simulink model "fft_filter"  (R2018a)
settings: Solver=VariableStepAuto  StartTime=0.0  StopTime=10  RelTol=1e-3
libraries: xbsIndex_r4 x6
settings Model: Creator=ESPINO NOTEBOOK  LastModifiedBy=ESPINO NOTEBOOK

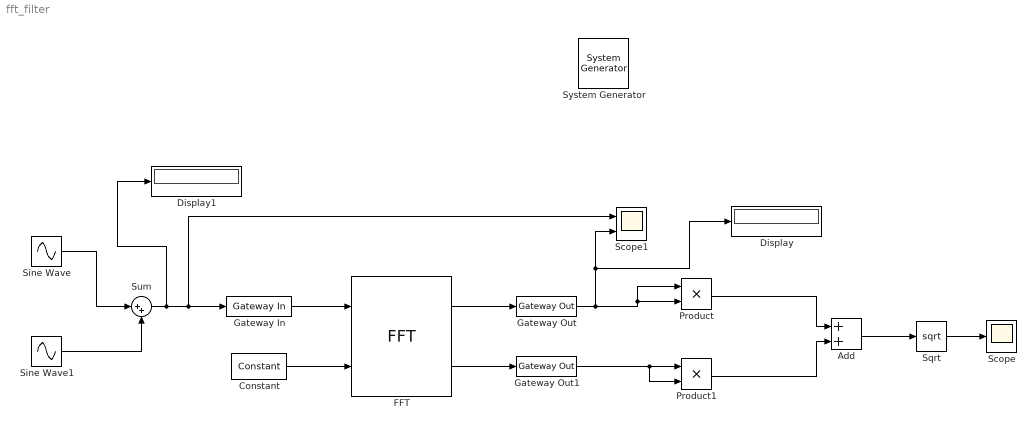
== system fft_filter ==
  " System Generator" : xbsIndex_r4/ System Generator  Tag=genX  xilinxfamily=zynq  part=xc7z020  speed=-2  package=clg400  synthesis_tool=Vivado  clock_wrapper=Clock Enables  directory=./netlist  proj_type=Vivado  Synth_file=Vivado Synthesis Defaults  Impl_file=Vivado Implementation Defaults  testbench=on  simulink_period=0.002  sysclk_period=10  dcm_input_clock_period=10  incr_netlist=off  trim_vbits=Everywhere in SubSystem  dbl_ovrd=According to Block Masks  core_generation=According to Block Masks  run_coregen=off  deprecated_control=off  eval_field=0  block_type=sysgen
  Add : Sum
  Constant : xbsIndex_r4/Constant  const=0  gui_display_data_type=Fixed-point  arith_type=Signed (2's comp)  n_bits=16  bin_pt=12  preci_type=Single  exp_width=8  frac_width=24  explicit_period=on  period=0.002  equ=P=C  opselect=C  inp2=PCIN>>17  opr=+  inp1=P  carry=CIN  dbl_ovrd=off  block_type=constant
  Display : Display
  Display1 : Display
  FFT : xbsIndex_r4/FFT  infoeditControl=Hardware notes: This block implements a burst IO radix-2 architecture if the <b><i>Optimize for</i></b> parameter is selected as <b><i>Resources</i></b>, and the input sample period is 8 times slower than the system sample period; otherwise a pipeline streaming architecture will be used.  transform_length=1024  scale_result_by_fft_length=off  bit_reversed_order=off  optimizegoal=Performance  start_frame=off  simulation_type=fast_sim  simulation_model=sysgen:ForwardFFT_Macro  latency=1  block_type=xfft_forward
  Gateway In : xbsIndex_r4/Gateway In  gui_display_data_type=Fixed-point  arith_type="Signed  (2's comp)"  n_bits=16  bin_pt=12  preci_type=Single  exp_width=8  frac_width=24  rows=1  columns=1  quantization=Truncate  overflow=Wrap  period=0.002  UseAsADC=off  ADCChannel='1'  interface=None  automatic_assignment=on  address_offset=hex2dec('00')  intf_name=''  intf_description=''  default_value=0  timing_constraint=None  locs_specified=off  LOCs={}  io_standard={}  inherit_from_input=off  hdl_port=on  dbl_ovrd=off  block_type=gatewayin
  Gateway Out : xbsIndex_r4/Gateway Out  inherit_from_input=off  hdl_port=on  rows=1  columns=1  UseAsDAC=off  DACChannel='1'  interface=None  automatic_assignment=on  address_offset=hex2dec('00')  intf_name=''  intf_description=''  timing_constraint=None  locs_specified=off  LOCs={}  io_standard={}  block_type=gatewayout
  Gateway Out1 : xbsIndex_r4/Gateway Out  inherit_from_input=off  hdl_port=on  rows=1  columns=1  UseAsDAC=off  DACChannel='1'  interface=None  automatic_assignment=on  address_offset=hex2dec('00')  intf_name=''  intf_description=''  timing_constraint=None  locs_specified=off  LOCs={}  io_standard={}  block_type=gatewayout
  Product : Product
  Product1 : Product
  Scope : Scope
  Scope1 : Scope  NumInputPorts=2
  Sine Wave : Sin  Frequency=2*pi*150  SampleTime=0
  Sine Wave1 : Sin  Frequency=2*pi*500  SampleTime=0
  Sqrt : Sqrt  SaturateOnIntegerOverflow=on
  Sum : Sum  Inputs=|++
  wires:
  Sine Wave/1 -> Sum/1
  Sine Wave1/1 -> Sum/2
  Sum/1 -> Display1/1, Scope1/1, Gateway In/1
  Gateway In/1 -> FFT/1
  Constant/1 -> FFT/2
  FFT/2 -> Gateway Out1/1
  FFT/1 -> Gateway Out/1
  Gateway Out1/1 -> Product1/2, Product1/1
  Gateway Out/1 -> Display/1, Scope1/2, Product/1, Product/2
  Product/1 -> Add/1
  Product1/1 -> Add/2
  Add/1 -> Sqrt/1
  Sqrt/1 -> Scope/1
